simulink model "recieve_udp"  (R2014b)
settings: Solver=ode3  StartTime=0.0  StopTime=inf  RelTol=1e-3
libraries: xpcutilitieslib x7, slrtlib x1
settings Model: SimulationMode=external  BufferReuse=off  Creator=Boreth  LastModifiedBy=Boreth
settings SolverCC: EnableConcurrentExecution=on
settings OptimizationCC: BlockReduction=off  OptimizeBlockIOStorage=off  BufferReuse=off  GlobalBufferReuse=off  ExpressionFolding=off  LocalBlockOutputs=off
settings HardwareCC: ProdIntDivRoundTo=Zero  ProdEndianess=LittleEndian  ProdLongLongMode=on  ProdHWDeviceType=Generic->32-bit x86 compatible
settings RTWCC: SystemTargetFile=slrt.tlc  TemplateMakefile=slrt_default_tmf  Description=Simulink Real-Time  ProcessScript=slrt_make_rtw_hook  RTWCompilerOptimization=On
settings SimulinkRealTimeCC: GeneratePreprocessorConditionals=Disable all  EnableShiftOperators=on

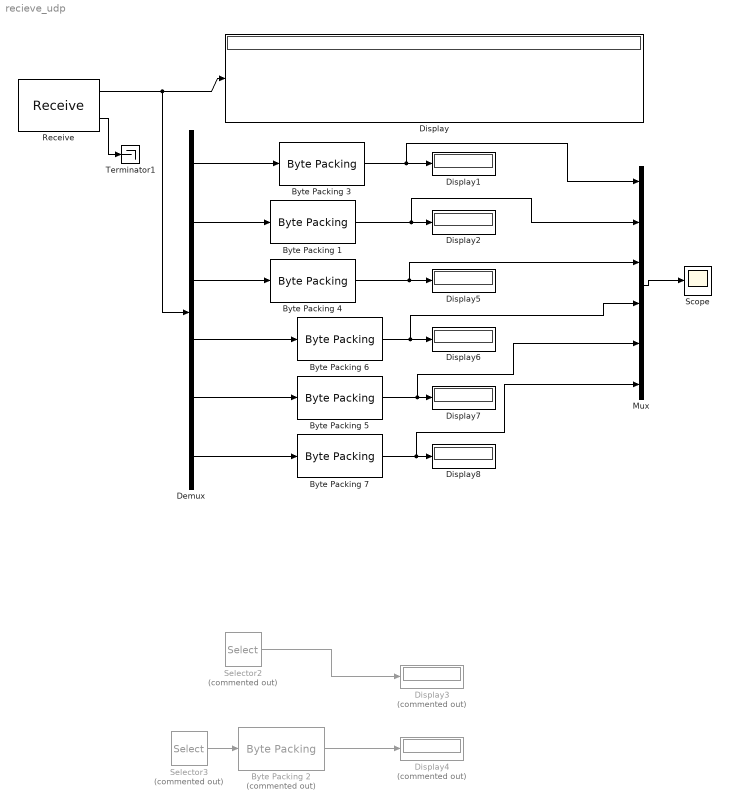
== system recieve_udp ==
  Byte Packing {1,3..7} (6 alike) : xpcutilitieslib/Byte Packing   MaskPackedDataType=single  MaskUnpackedDataTypes={'uint8'}  MaskAlignment=4
  Byte Packing 2 : xpcutilitieslib/Byte Packing   Commented=on  MaskPackedDataType=single  MaskUnpackedDataTypes={'uint8'}  MaskAlignment=4
  Demux : Demux  Outputs=[4 4 4 4 4 4]
  Display{,1..2,5..8} (7 alike) : Display
  Display3 : Display  Commented=on
  Display4 : Display  Commented=on
  Mux : Mux  Inputs=6
  "Receive " : slrtlib/UDP/Receive   ipAddress=192.168.1.100  ipPort=50002  width=24  vblLen=on  sampletime=0.05
  Scope : Scope
  Selector2 : Selector  Commented=on  InputPortWidth=5
  Selector3 : Selector  Commented=on  InputPortWidth=5  Indices=[2:5]
  Terminator1 : Terminator
  wires:
  "Receive "/2 -> Terminator1/1
  "Receive "/1 -> Display/1, Demux/1
  Byte Packing 1/1 -> Mux/2, Display2/1
  Demux/1 -> Byte Packing 3/1
  Demux/2 -> Byte Packing 1/1
  ? -> Selector3/1
  ? -> Selector2/1
  Byte Packing 2/1 -> Display4/1
  Selector2/1 -> Display3/1
  Selector3/1 -> Byte Packing 2/1
  Byte Packing 3/1 -> Mux/1, Display1/1
  Byte Packing 4/1 -> Mux/3, Display5/1
  Demux/3 -> Byte Packing 4/1
  Byte Packing 5/1 -> Mux/5, Display7/1
  Demux/4 -> Byte Packing 6/1
  Demux/5 -> Byte Packing 5/1
  Byte Packing 6/1 -> Mux/4, Display6/1
  Byte Packing 7/1 -> Mux/6, Display8/1
  Demux/6 -> Byte Packing 7/1
  Mux/1 -> Scope/1
